simulink subsystem "ins"  (R2024b)
settings: Solver=VariableStepAuto  StartTime=0.0  StopTime=10.0  RelTol=1e-3
settings Model: Creator=yagiz  LastModifiedBy=yagiz

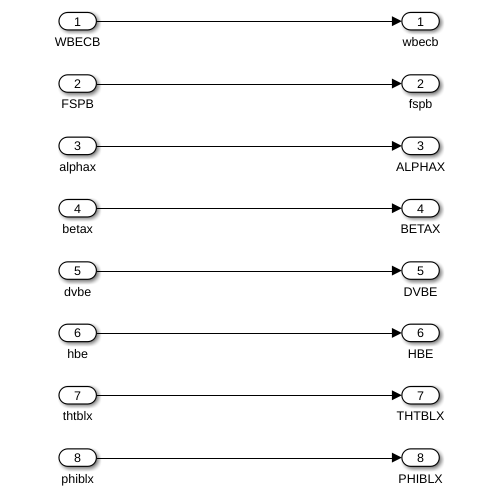
[thumbnail: Simulink's stored preview of the top-level diagram]
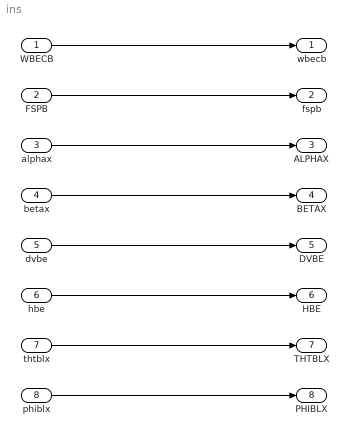
== system ins ==
  WBECB : Inport
  FSPB : Inport  Port=2
  alphax : Inport  Port=3
  betax : Inport  Port=4
  dvbe : Inport  Port=5
  hbe : Inport  Port=6
  thtblx : Inport  Port=7
  phiblx : Inport  Port=8
  wbecb : Outport
  fspb : Outport  Port=2
  ALPHAX : Outport  Port=3
  BETAX : Outport  Port=4
  DVBE : Outport  Port=5
  HBE : Outport  Port=6
  THTBLX : Outport  Port=7
  PHIBLX : Outport  Port=8
  wires:
  WBECB/1 -> wbecb/1
  FSPB/1 -> fspb/1
  alphax/1 -> ALPHAX/1
  betax/1 -> BETAX/1
  dvbe/1 -> DVBE/1
  hbe/1 -> HBE/1
  thtblx/1 -> THTBLX/1
  phiblx/1 -> PHIBLX/1
